simulink model "mixed"  (R2021a)
settings: Solver=VariableStepAuto  StartTime=0.0  StopTime=100  RelTol=1e-3
undefined symbols (not defined in the file): C, r
settings Model: Creator=user  LastModifiedBy=lenovo
settings SolverCC: AlgebraicLoopSolver=TrustRegion
settings DebuggingCC: SFMachineParentedDataDiag=warning
settings SFSimCC: CustomCodeUndefinedFunction=UseInterfaceOnly

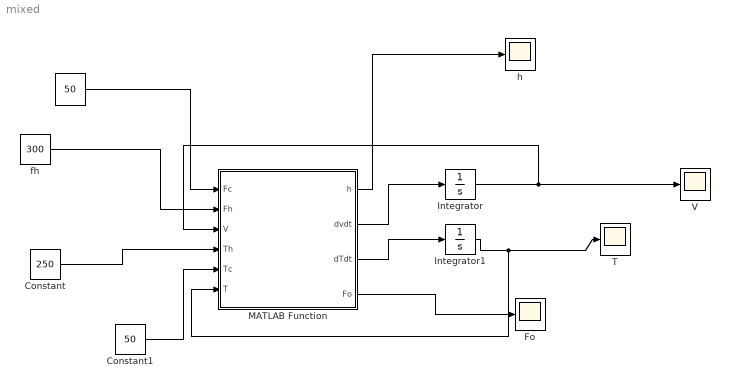
== system mixed ==
  " " : Constant  Value=50
  Constant : Constant  Value=250
  Constant1 : Constant  Value=50
  Fo : Scope
  Integrator : Integrator  InitialCondition=100
  Integrator1 : Integrator  InitialCondition=200
  MATLAB Function : MATLAB Function  TreatAsAtomicUnit=on
  T : Scope
  V : Scope
  fh : Constant  Value=300
  h : Scope
  wires:
  fh/1 -> MATLAB Function/2(Fh)
  " "/1 -> MATLAB Function/1(Fc)
  Constant/1 -> MATLAB Function/4(Th)
  Constant1/1 -> MATLAB Function/5(Tc)
  MATLAB Function/3(dTdt) -> Integrator1/1
  Integrator/1 -> MATLAB Function/3(V), V/1
  Integrator1/1 -> MATLAB Function/6(T), T/1
  MATLAB Function/4(Fo) -> Fo/1
  MATLAB Function/2(dvdt) -> Integrator/1
  MATLAB Function/1(h) -> h/1

== matlab function mixed/MATLAB Function ==
  data: Fc input; Fh input; V input; Th input; Tc input; T input; h output; dvdt output; dTdt output; Fo output; r parameter; C parameter
function [h, dvdt, dTdt, Fo] =mixed(Fc, Fh, V, Th, Tc, T, r, C)

A=pi*r*r;

h=V/A;

Fo=C*sqrt(h);

dvdt=(Fh+Fc)-Fo;

dTdt=((Fh*(Th-T))/(V))+((Fc*(Tc-T))/(V));

end
